simulink model "Copy_of_Quad_Nonlinear_Pitch_OL"  (R2020a)
settings: Solver=ode4  StartTime=0.0  StopTime=15  FixedStep=0.01  RelTol=1e-3
InitFcn:
  | QuadParameter
values from neighbouring files (symbols this model uses):
  b = 1.10794e-5    (= 1.10794e-05)    [QuadParameter.m]    (also in QuadParameter_v1.m = 3.13e-05; Scenario_I.mat = 3.13e-05; pitch_pameterestimation_result.m = 1.30238026482e-05; result_J.m = SDOSessionData.Data.Workspace.LocalWorkspace.EstimatedParams)
  d_cg = 0.2    [QuadParameter.m]    (also in QuadParameter_v1.m; pitch_pameterestimation_result.m = 0.251635071944)
  g = 9.81    [QuadParameter.m]
  h_cg = 0.02    [QuadParameter.m]    (also in pitch_pameterestimation_result.m = 0.0335128405392)
  J_yy = 0.03066    [QuadParameter.m]    (also in pitch_pameterestimation_result.m = 0.142533306975; pitch_parameter_estiation_result.m = 0.179530810307)
  m2 = 1.074    [QuadParameter.m]
  m_tot = 1.074    [QuadParameter.m]
  miu_k = 0.002    [QuadParameter.m]    (also in pitch_pameterestimation_result.m = 1.39726024883e-05)
  r_y = 0.01    [QuadParameter.m]    (also in pitch_pameterestimation_result.m = 6.80104645207e-05)
undefined symbols (not defined in the file or in its folder): AHRS_RCP, magnitude
settings Model: OrderedModelArguments=off  Creator=Ali  LastModifiedBy=Ali

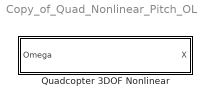
== system Copy_of_Quad_Nonlinear_Pitch_OL ==
  Quadcopter 3DOF Nonlinear : Subsystem  TreatAsAtomicUnit=on
  wires:
  ? -> Quadcopter 3DOF Nonlinear/1(Omega)

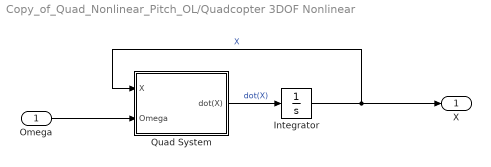
== system Copy_of_Quad_Nonlinear_Pitch_OL/Quadcopter 3DOF Nonlinear ==
  Omega : Inport
  Integrator : Integrator  InitialCondition=AHRS_RCP(1, :)
  Quad System : Subsystem
  X : Outport
  wires:
  Integrator/1 -> Quad System/1(X), X/1  "X"
  Quad System/1(dot(X)) -> Integrator/1  "dot(X)"
  Omega/1 -> Quad System/2(Omega)

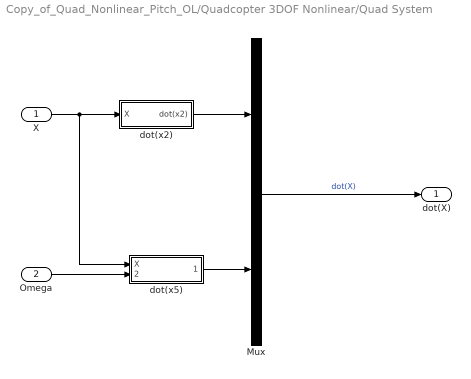
== system Copy_of_Quad_Nonlinear_Pitch_OL/Quadcopter 3DOF Nonlinear/Quad System ==
  X : Inport
  Omega : Inport  Port=2
  Mux : Mux  Inputs=2
  dot(x2) : Subsystem
  dot(x5) : Subsystem
  dot(X) : Outport
  wires:
  Mux/1 -> dot(X)/1  "dot(X)"
  dot(x2)/1(dot(x2)) -> Mux/1
  dot(x5)/1(dot(x5)) -> Mux/2
  X/1 -> dot(x5)/1(X), dot(x2)/1(X)
  Omega/1 -> dot(x5)/2(Omega)

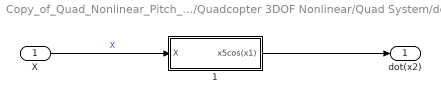
== system Copy_of_Quad_Nonlinear_Pitch_OL/Quadcopter 3DOF Nonlinear/Quad System/dot(x2) ==
  X : Inport
  1 : Subsystem
  dot(x2) : Outport
  wires:
  X/1 -> 1/1(X)  "X"
  1/1(x5cos(x1)) -> dot(x2)/1

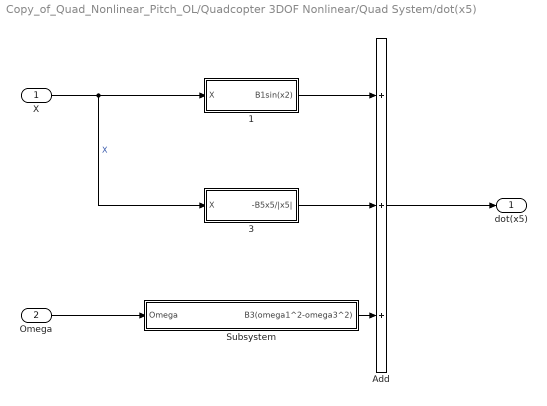
== system Copy_of_Quad_Nonlinear_Pitch_OL/Quadcopter 3DOF Nonlinear/Quad System/dot(x5) ==
  X : Inport
  Omega : Inport  Port=2
  1 : Subsystem
  3 : Subsystem
  Add : Sum  Inputs=+++
  Subsystem : Subsystem
  dot(x5) : Outport
  wires:
  X/1 -> 3/1(X), 1/1(X)  "X"
  Omega/1 -> Subsystem/1(Omega)
  Add/1 -> dot(x5)/1
  Subsystem/1(B3(omega1^2-omega3^2)) -> Add/3
  3/1("-B5x5/|x5| ") -> Add/2
  1/1(B1sin(x2)) -> Add/1

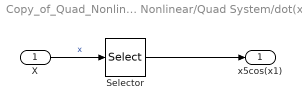
== system Copy_of_Quad_Nonlinear_Pitch_OL/Quadcopter 3DOF Nonlinear/Quad System/dot(x2)/1 ==
  X : Inport
  Selector : Selector  InputPortWidth=2  IndexOptions=Index vector (dialog)  Indices=[2]  OutputSizes=1
  x5cos(x1) : Outport
  wires:
  X/1 -> Selector/1  "x"
  Selector/1 -> x5cos(x1)/1

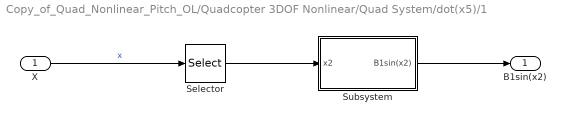
== system Copy_of_Quad_Nonlinear_Pitch_OL/Quadcopter 3DOF Nonlinear/Quad System/dot(x5)/1 ==
  X : Inport
  Selector : Selector  InputPortWidth=2  IndexOptions=Index vector (dialog)  Indices=[1]  OutputSizes=1
  Subsystem : Subsystem
  B1sin(x2) : Outport
  wires:
  X/1 -> Selector/1  "x"
  Subsystem/1(B1sin(x2)) -> B1sin(x2)/1
  Selector/1 -> Subsystem/1(x2)

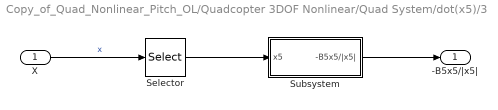
== system Copy_of_Quad_Nonlinear_Pitch_OL/Quadcopter 3DOF Nonlinear/Quad System/dot(x5)/3 ==
  X : Inport
  Selector : Selector  InputPortWidth=2  IndexOptions=Index vector (dialog)  Indices=[2]  OutputSizes=1
  Subsystem : Subsystem
  "-B5x5/|x5| " : Outport
  wires:
  X/1 -> Selector/1  "x"
  Subsystem/1("-B5x5/|x5| ") -> "-B5x5/|x5| "/1
  Selector/1 -> Subsystem/1(x5)

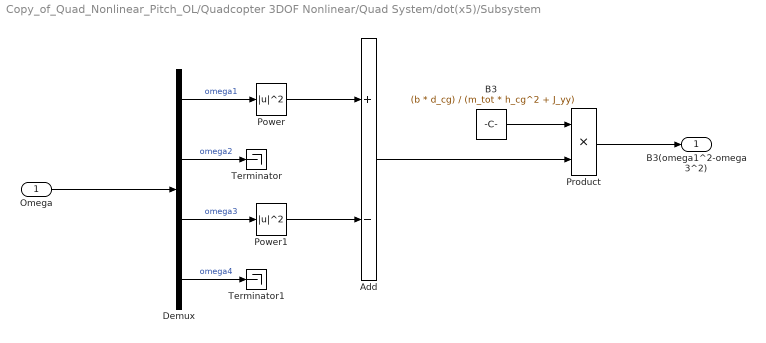
== system Copy_of_Quad_Nonlinear_Pitch_OL/Quadcopter 3DOF Nonlinear/Quad System/dot(x5)/Subsystem ==
  Omega : Inport
  Add : Sum  Inputs=+-
  B3 : Constant  Value=(b * d_cg) / (m_tot * h_cg^2 + J_yy)
  Demux : Demux
  Power : Math  Operator=magnitude^2  SaturateOnIntegerOverflow=on
  Power1 : Math  Operator=magnitude^2  SaturateOnIntegerOverflow=on
  Product : Product
  Terminator : Terminator
  Terminator1 : Terminator
  B3(omega1^2-omega3^2) : Outport
  wires:
  Product/1 -> B3(omega1^2-omega3^2)/1
  Power1/1 -> Add/2
  Add/1 -> Product/2
  Power/1 -> Add/1
  B3/1 -> Product/1
  Omega/1 -> Demux/1
  Demux/3 -> Power1/1  "omega3"
  Demux/1 -> Power/1  "omega1"
  Demux/2 -> Terminator/1  "omega2"
  Demux/4 -> Terminator1/1  "omega4"

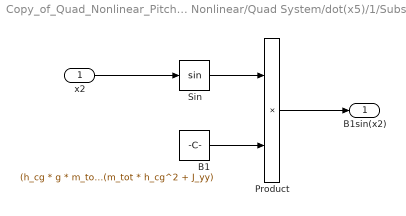
== system Copy_of_Quad_Nonlinear_Pitch_OL/Quadcopter 3DOF Nonlinear/Quad System/dot(x5)/1/Subsystem ==
  x2 : Inport
  B1 : Constant  Value=(h_cg * g * m_tot) / (m_tot * h_cg^2 + J_yy)
  Product : Product
  Sin : Trigonometry
  B1sin(x2) : Outport
  wires:
  Product/1 -> B1sin(x2)/1
  x2/1 -> Sin/1
  B1/1 -> Product/2
  Sin/1 -> Product/1

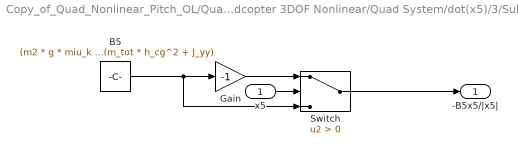
== system Copy_of_Quad_Nonlinear_Pitch_OL/Quadcopter 3DOF Nonlinear/Quad System/dot(x5)/3/Subsystem ==
  x5 : Inport
  B5 : Constant  Value=(m2 * g * miu_k * r_y) / (m_tot * h_cg^2 + J_yy)
  Gain : Gain  Gain=-1
  Switch : Switch  Criteria=u2 > Threshold
  "-B5x5/|x5| " : Outport
  wires:
  Switch/1 -> "-B5x5/|x5| "/1
  B5/1 -> Switch/3, Gain/1
  x5/1 -> Switch/2
  Gain/1 -> Switch/1
